simulink model "MAIN_V4"  (R2022a)
settings: Solver=VariableStepAuto  StartTime=0.0  StopTime=10  RelTol=1e-3
undefined symbols (not defined in the file): angDrag, c_Fuel, CM_FUEL_b, cmFuel_cmL, g, k_Fuel, KX, KY, L_TV, linDrag, m_dot, m_iFuel, VRfromNED_cordT, W_LANDER
libraries: matrix_library x4, slpidlib x1, dspsrcs4 x1, shared6dof x1, aerolibanim x1, simulink_extras x1, vrlib x1
settings Model: Creator=josepfamador  LastModifiedBy=Siste
settings DebuggingCC: UnconnectedInputMsg=warning  UnconnectedOutputMsg=warning  UnconnectedLineMsg=warning
settings RTWCC: DLArmComputeVersion=19.05

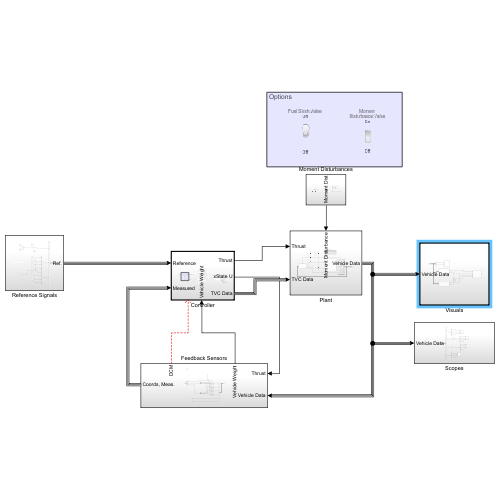
[thumbnail: Simulink's stored preview of the top-level diagram]
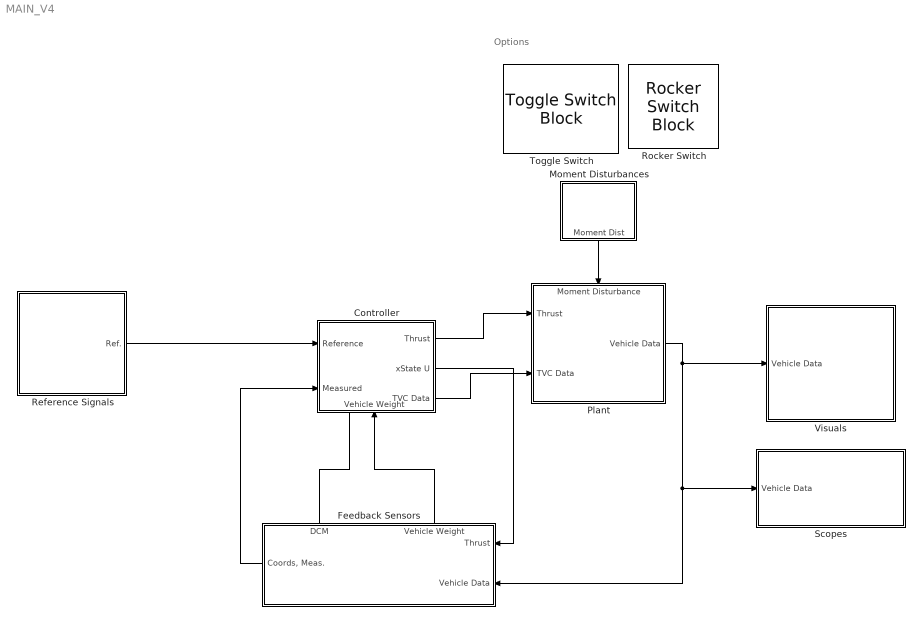
== system MAIN_V4 ==
  note: Options
  Controller : Subsystem  TreatAsAtomicUnit=on
      settings: PortSchema="{\"entries\":[{\"content\":{\"sides\":[{\"content\":{\"connectorIds\":[\"In1\",\"In2\"]},\"type\":\"ConnectorPlacement.EquallySpacedRectSide\",\"uuid\":\"a9e81047-82e7-465f-ace1-8f718b90561e\"},{\"content\":{\"connectorIds\":[\"Out1\",\"Out2\",\"Out3\"],\"side\":\"RIGHT\"},\"type\":\"ConnectorPlacement.EquallySpacedRectSide\",\"uuid\":\"e48627af-c2aa-4531-b804-41f44ff16765\"},{\"content\":{\"connectorIds\":[],\"side\":\"TOP\"},\"type\":\"ConnectorPlacement.EquallySpacedRectSide\",\"uuid\":\"f9e16229-b89b-4f8f-8331-a0f549979ea4\"},{\"content\":{\"connectorIds\":[\"In3\"],\"side\":\"BOTTOM\"},\"type\":\"ConnectorPlacement.EquallySpacedRectSide\",\"uuid\":\"04cdfde2-d4f0-49a2-8a73-ed462fcd7361\"}]},\"type\":\"ConnectorPlacement.EquallySpacedConnector\",\"uuid\":\"554d82b7-b70e-4d8b-909f-79f77f042d74\"}],\"packageUris\":[\"http://schema.mathworks.com/mf0/Connector/R2020b\"],\"version\":\"1.0\"}"
  Feedback Sensors : Subsystem
      settings: PortSchema="{\"entries\":[{\"content\":{\"sides\":[{\"content\":{\"connectorIds\":[\"In1\",\"In2\"]},\"type\":\"ConnectorPlacement.EquallySpacedRectSide\",\"uuid\":\"d175d4a2-8e54-4a4e-8022-790f4682ab06\"},{\"content\":{\"connectorIds\":[\"Out1\"],\"side\":\"RIGHT\"},\"type\":\"ConnectorPlacement.EquallySpacedRectSide\",\"uuid\":\"24f1a27c-01cc-42b0-9970-402e35771ac9\"},{\"content\":{\"connectorIds\":[\"Out2\",\"Out3\"],\"side\":\"TOP\"},\"type\":\"ConnectorPlacement.EquallySpacedRectSide\",\"uuid\":\"3106a051-6715-4641-97e9-232ad93b76cc\"}]},\"type\":\"ConnectorPlacement.EquallySpacedConnector\",\"uuid\":\"a13f3672-a567-4503-9f3c-ec2ff34e4e5d\"}],\"packageUris\":[\"http://schema.mathworks.com/mf0/Connector/R2020b\"],\"version\":\"1.0\"}"
  Moment Disturbances : Subsystem
  Plant : Subsystem
      settings: PortSchema="{\"entries\":[{\"content\":{\"sides\":[{\"content\":{\"connectorIds\":[\"In1\",\"In2\"]},\"type\":\"ConnectorPlacement.EquallySpacedRectSide\",\"uuid\":\"a9e81047-82e7-465f-ace1-8f718b90561e\"},{\"content\":{\"connectorIds\":[\"Out1\"],\"side\":\"RIGHT\"},\"type\":\"ConnectorPlacement.EquallySpacedRectSide\",\"uuid\":\"e48627af-c2aa-4531-b804-41f44ff16765\"},{\"content\":{\"connectorIds\":[\"In3\"],\"side\":\"TOP\"},\"type\":\"ConnectorPlacement.EquallySpacedRectSide\",\"uuid\":\"f9e16229-b89b-4f8f-8331-a0f549979ea4\"}]},\"type\":\"ConnectorPlacement.EquallySpacedConnector\",\"uuid\":\"554d82b7-b70e-4d8b-909f-79f77f042d74\"}],\"packageUris\":[\"http://schema.mathworks.com/mf0/Connector/R2020b\"],\"version\":\"1.0\"}"
  Reference Signals : Subsystem
  Rocker Switch : RockerSwitchBlock
      settings: Values={{'Off', 'On'}, [0 1]}
  Scopes : Subsystem
  Toggle Switch : ToggleSwitchBlock
      settings: Values={{'Off', 'On'}, [0 1]}
  Visuals : Subsystem  TreatAsAtomicUnit=on
  wires:
  Moment Disturbances/1(Moment Dist) -> Plant/3(Moment Disturbance)
  Plant/1(Vehicle Data) -> Scopes/1(Vehicle Data), Feedback Sensors/2(Vehicle Data), Visuals/1(Vehicle Data)
  Controller/1(Thrust) -> Plant/1(Thrust)
  Feedback Sensors/2(Vehicle Weight) -> Controller/3(Vehicle Weight)
  Feedback Sensors/3(DCM) -> ?
  Reference Signals/1(Ref.) -> Controller/1(Reference)
  Controller/2(xState U) -> Feedback Sensors/1(Thrust)
  Feedback Sensors/1("Coords, Meas.") -> Controller/2(Measured)
  Controller/3(TVC Data) -> Plant/2(TVC Data)

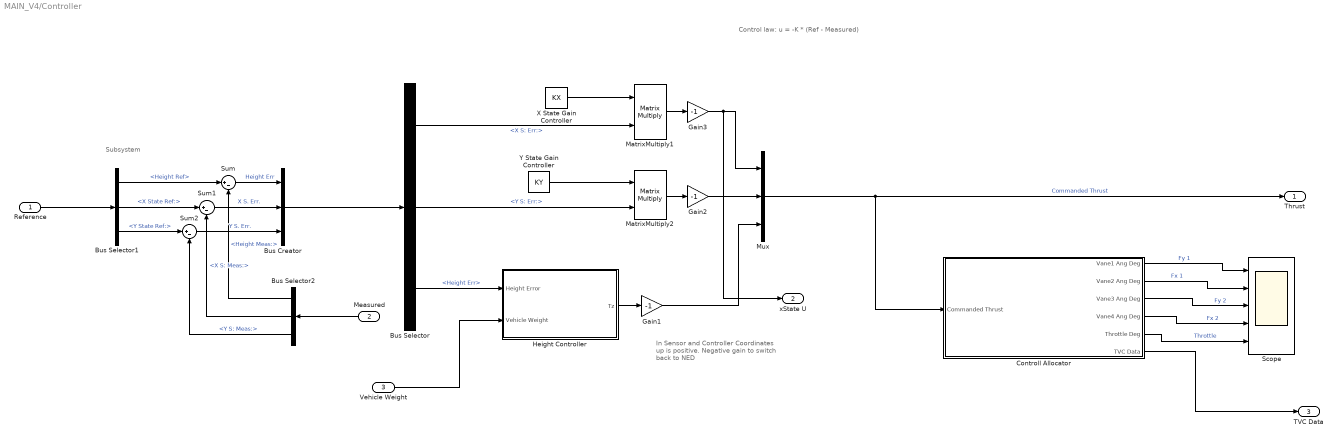
== system MAIN_V4/Controller ==
  note: Subsystem
  note: Control law: u = -K * (Ref - Measured)
  note: In Sensor and Controller Coordinates up is positive. Negative gain to switch back to NED
  Reference : Inport
  Measured : Inport  Port=2
  Vehicle Weight : Inport  Port=3
  Bus Creator : BusCreator  Inputs=3
  Bus Selector : BusSelector  OutputSignals=X S: Err:,Y S: Err:,Height Err
  Bus Selector1 : BusSelector  OutputSignals=Height Ref,X State Ref:,Y State Ref:
  Bus Selector2 : BusSelector  OutputSignals=Height Meas:,X S: Meas:,Y S: Meas:
  Controll Allocator : Subsystem
  Gain1 : Gain  Gain=-1
  Gain2 : Gain  Gain=-1
  Gain3 : Gain  Gain=-1
  Height Controller : Subsystem
  MatrixMultiply1 : Product  Multiplication=Matrix(*)
  MatrixMultiply2 : Product  Multiplication=Matrix(*)
  Mux : Mux  Inputs=3
  Scope : Scope  NumInputPorts=5
  Sum : Sum  Inputs=|+-
  Sum1 : Sum  Inputs=|+-
  Sum2 : Sum  Inputs=|+-
  X State Gain Controller : Constant  Value=KX  VectorParams1D=off
  Y State Gain Controller : Constant  Value=KY  VectorParams1D=off
  Thrust : Outport
  xState U : Outport  Port=2
  TVC Data : Outport  Port=3
  wires:
  Vehicle Weight/1 -> Height Controller/2(Vehicle Weight)
  Height Controller/1(Tz) -> Gain1/1
  Mux/1 -> Controll Allocator/1(Commanded Thrust), Thrust/1  "Commanded Thrust"
  Gain1/1 -> Mux/3
  X State Gain Controller/1 -> MatrixMultiply1/1
  Bus Selector/1 -> MatrixMultiply1/2  "<X S: Err:>"
  Y State Gain Controller/1 -> MatrixMultiply2/1
  Bus Selector/2 -> MatrixMultiply2/2  "<Y S: Err:>"
  Bus Selector/3 -> Height Controller/1(Height Error)  "<Height Err>"
  MatrixMultiply2/1 -> Gain2/1
  MatrixMultiply1/1 -> Gain3/1
  Gain2/1 -> Mux/2
  Gain3/1 -> xState U/1, Mux/1
  Controll Allocator/1(Vane1 Ang Deg) -> Scope/1  "Fy 1"
  Controll Allocator/2(Vane2 Ang Deg) -> Scope/2  "Fx 1"
  Controll Allocator/3(Vane3 Ang Deg) -> Scope/3  "Fy 2"
  Controll Allocator/4(Vane4 Ang Deg) -> Scope/4  "Fx 2"
  Controll Allocator/5(Throttle Deg) -> Scope/5  "Throttle"
  Reference/1 -> Bus Selector1/1
  Bus Selector2/2 -> Sum1/2  "<X S: Meas:>"
  Sum1/1 -> Bus Creator/2  "X S. Err."
  Sum2/1 -> Bus Creator/3  "Y S. Err."
  Bus Selector1/2 -> Sum1/1  "<X State Ref:>"
  Sum/1 -> Bus Creator/1  "Height Err"
  Bus Selector2/3 -> Sum2/2  "<Y S: Meas:>"
  Bus Selector1/3 -> Sum2/1  "<Y State Ref:>"
  Bus Selector1/1 -> Sum/1  "<Height Ref>"
  Bus Creator/1 -> Bus Selector/1
  Bus Selector2/1 -> Sum/2  "<Height Meas:>"
  Measured/1 -> Bus Selector2/1
  Controll Allocator/6(TVC Data) -> TVC Data/1

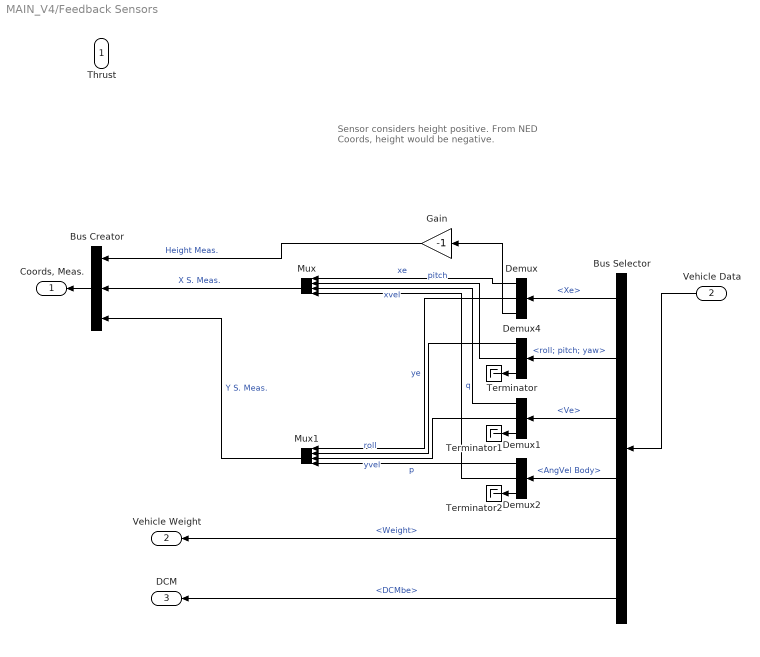
== system MAIN_V4/Feedback Sensors ==
  note: Sensor considers height positive.
      | From NED Coords, height would be negative.
  Thrust : Inport
  Vehicle Data : Inport  Port=2
  Bus Creator : BusCreator  Inputs=3
  Bus Selector : BusSelector  OutputSignals=Xe,roll; pitch; yaw,Ve,AngVel Body,Weight,DCMbe
  Demux{,1..2,4} (4 alike) : Demux  Outputs=3
  Gain : Gain  Gain=-1
  Mux : Mux
  Mux1 : Mux
  Terminator : Terminator
  Terminator1 : Terminator
  Terminator2 : Terminator
  "Coords, Meas." : Outport
  Vehicle Weight : Outport  Port=2
  DCM : Outport  Port=3
  wires:
  Vehicle Data/1 -> Bus Selector/1
  Bus Selector/1 -> Demux/1  "<Xe>"
  Bus Selector/2 -> Demux4/1  "<roll; pitch; yaw>"
  Demux/3 -> Gain/1
  Demux/1 -> Mux/1  "xe"
  Demux/2 -> Mux1/1  "ye"
  Gain/1 -> Bus Creator/1  "Height Meas."
  Bus Selector/5 -> Vehicle Weight/1  "<Weight>"
  Bus Selector/6 -> DCM/1  "<DCMbe>"
  Demux4/2 -> Mux/2  "pitch"
  Bus Selector/4 -> Demux2/1  "<AngVel Body>"
  Bus Selector/3 -> Demux1/1  "<Ve>"
  Demux1/1 -> Mux/3  "xvel"
  Demux2/2 -> Mux/4  "q"
  Mux/1 -> Bus Creator/2  "X S. Meas."
  Mux1/1 -> Bus Creator/3  "Y S. Meas."
  Demux4/1 -> Mux1/2  "roll"
  Demux1/2 -> Mux1/3  "yvel"
  Demux2/1 -> Mux1/4  "p"
  Demux4/3 -> Terminator/1
  Demux1/3 -> Terminator1/1
  Demux2/3 -> Terminator2/1
  Bus Creator/1 -> "Coords, Meas."/1

== system MAIN_V4/Moment Disturbances ==
  Demux : Demux  Outputs=3
  Disturbance Vector : Subsystem
  Moment Disturbance : Constant  Value=0
  Scope : Scope  NumInputPorts=3
  Slider : SliderBlock  ScaleMax=20
  Moment Dist : Outport
  wires:
  Disturbance Vector/1(Out1) -> Demux/1, Moment Dist/1
  Moment Disturbance/1 -> Disturbance Vector/Enable
  Demux/1 -> Scope/1
  Demux/2 -> Scope/2
  Demux/3 -> Scope/3

== system MAIN_V4/Plant ==
  note: Coordinate Frame used.
      | X
      | Into the Screen. Away from Observer
      |
      | Y
      | Right Of Screen. Observer's Right
      |
      | Z
      | Down to ground. Observer's Ground
  Thrust : Inport
  TVC Data : Inport  Port=2
  Moment Disturbance : Inport  Port=3
  6DOF (Euler Angles) : shared6dof/6DOF (Euler Angles)  units=Metric (MKS)  mtype=Fixed  rep=Euler Angles  xme_0=[0 0 0]  Vm_0=[0 0 0]  eul_0=[0 0 0]  pm_0=[0 0 0]  mass_0=M_lander  mass_e=0.5  mass_f=2.0  inertia=I  inertia_e=eye(3)  inertia_f=2*eye(3)  k_quat=1.0  vre_flag=on  abi_flag=off  aMode=0  xme_statename=''  Vm_statename=''  eul_statename=''  quat_statename=''  pm_statename=''  mass_statename=''
      settings: SourceProductBaseCode=AE,PW,DR,MT,VE
  Bus Creator1 : BusCreator  Inputs=11
  Forces and Moments : Subsystem
      settings: PortSchema="{\"entries\":[{\"content\":{\"sides\":[{\"content\":{\"connectorIds\":[\"In1\"]},\"type\":\"ConnectorPlacement.EquallySpacedRectSide\",\"uuid\":\"828f15e3-cbad-415f-85fb-ba6a8e0cd3b9\"},{\"content\":{\"connectorIds\":[\"Out1\",\"Out2\",\"Out3\"],\"side\":\"RIGHT\"},\"type\":\"ConnectorPlacement.EquallySpacedRectSide\",\"uuid\":\"5000816a-8e0b-4f65-bf77-7d05076903d9\"},{\"content\":{\"connectorIds\":[\"In2\"],\"side\":\"TOP\"},\"type\":\"ConnectorPlacement.EquallySpacedRectSide\",\"uuid\":\"57f53c13-0af9-4c97-9cf0-1ba4f356b699\"}]},\"type\":\"ConnectorPlacement.EquallySpacedConnector\",\"uuid\":\"7fdc047f-04f4-4b62-afef-380f9e9b929b\"}],\"packageUris\":[\"http://schema.mathworks.com/mf0/Connector/R2020b\"],\"version\":\"1.0\"}"
  Sum : Sum  Inputs=++|
  Sum1 : Sum  Inputs=++|
  Vehicle Data : Outport
  wires:
  6DOF (Euler Angles)/7 -> Bus Creator1/7  "AngAcc body"
  6DOF (Euler Angles)/3 -> Bus Creator1/3  "roll, pitch, yaw"
  Sum/1 -> 6DOF (Euler Angles)/1
  Thrust/1 -> Sum/1, Forces and Moments/2(Thrust), Bus Creator1/10  "Thrust"
  6DOF (Euler Angles)/4 -> Bus Creator1/4  "DCMbe"
  Forces and Moments/1(SumF) -> Sum/2
  Forces and Moments/2(Moments) -> Sum1/2
  6DOF (Euler Angles)/6 -> Bus Creator1/6  "AngVel Body"
  6DOF (Euler Angles)/1 -> Bus Creator1/1  "Ve"
  6DOF (Euler Angles)/2 -> Bus Creator1/2  "Xe"
  6DOF (Euler Angles)/5 -> Bus Creator1/5  "Vb"
  6DOF (Euler Angles)/8 -> Bus Creator1/8  "Acc Body"
  Bus Creator1/1 -> Forces and Moments/1(Vehicle Data), Vehicle Data/1
  Sum1/1 -> 6DOF (Euler Angles)/2
  Moment Disturbance/1 -> Sum1/1
  Forces and Moments/3(Total Weight) -> Bus Creator1/9  "Weight"
  TVC Data/1 -> Bus Creator1/11  "TVC Data"

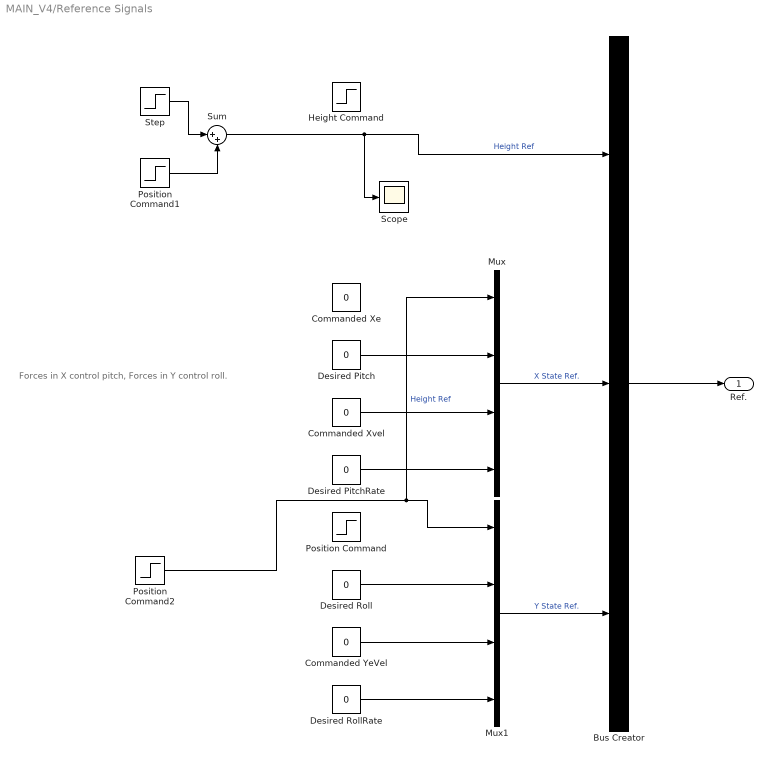
== system MAIN_V4/Reference Signals ==
  note: Forces in X control pitch, Forces in Y control roll.
  Bus Creator : BusCreator  Inputs=3
  Commanded Xe : Constant  Value=0
  Commanded Xvel : Constant  Value=0
  Commanded YeVel : Constant  Value=0
  Desired Pitch : Constant  Value=0
  Desired PitchRate : Constant  Value=0
  Desired Roll : Constant  Value=0
  Desired RollRate : Constant  Value=0
  Height Command : Step  SampleTime=0
  Mux : Mux
  Mux1 : Mux
  Position Command : Step  Time=3  SampleTime=0
  Position Command1 : Step  Time=0.5  SampleTime=0
  Position Command2 : Step  SampleTime=0
  Scope : Scope
  Step : Step  Time=6  After=-1  SampleTime=0
  Sum : Sum  Inputs=|++
  Ref. : Outport
  wires:
  Sum/1 -> Scope/1, Bus Creator/1  "Height Ref"
  Desired PitchRate/1 -> Mux/4
  Commanded Xvel/1 -> Mux/3
  Desired Pitch/1 -> Mux/2
  Mux/1 -> Bus Creator/2  "X State Ref."
  Desired Roll/1 -> Mux1/2
  Commanded YeVel/1 -> Mux1/3
  Desired RollRate/1 -> Mux1/4
  Mux1/1 -> Bus Creator/3  "Y State Ref."
  Bus Creator/1 -> Ref./1
  Position Command1/1 -> Sum/2
  Step/1 -> Sum/1
  Position Command2/1 -> Mux/1, Mux1/1  "Height Ref"

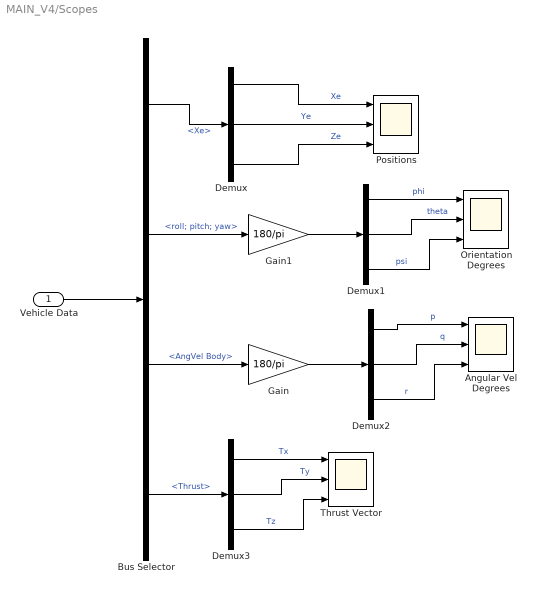
== system MAIN_V4/Scopes ==
  Vehicle Data : Inport
  Angular Vel Degrees : Scope  NumInputPorts=3
  Bus Selector : BusSelector  OutputSignals=Xe,roll; pitch; yaw,AngVel Body,Thrust
  Demux{,1..3} (4 alike) : Demux  Outputs=3
  Gain : Gain  Gain=180/pi
  Gain1 : Gain  Gain=180/pi
  Orientation Degrees : Scope  NumInputPorts=3
  Positions : Scope  NumInputPorts=3
  Thrust Vector : Scope  NumInputPorts=3
  wires:
  Vehicle Data/1 -> Bus Selector/1
  Bus Selector/1 -> Demux/1  "<Xe>"
  Bus Selector/3 -> Gain/1  "<AngVel Body>"
  Bus Selector/2 -> Gain1/1  "<roll; pitch; yaw>"
  Demux/2 -> Positions/2  "Ye"
  Demux/1 -> Positions/1  "Xe"
  Demux/3 -> Positions/3  "Ze"
  Demux1/1 -> Orientation Degrees/1  "phi"
  Demux1/2 -> Orientation Degrees/2  "theta"
  Demux1/3 -> Orientation Degrees/3  "psi"
  Demux2/2 -> Angular Vel Degrees/2  "q"
  Demux2/1 -> Angular Vel Degrees/1  "p"
  Demux2/3 -> Angular Vel Degrees/3  "r"
  Bus Selector/4 -> Demux3/1  "<Thrust>"
  Demux3/1 -> Thrust Vector/1  "Tx"
  Demux3/2 -> Thrust Vector/2  "Ty"
  Demux3/3 -> Thrust Vector/3  "Tz"
  Gain/1 -> Demux2/1
  Gain1/1 -> Demux1/1

== system MAIN_V4/Visuals ==
  Vehicle Data : Inport
  6DoF Animation1 : aerolibanim/6DoF Animation  u1=[-5 5 -5 5 0 4]  u2=0.1  u3=1  u4=[0 0 -1]  u5=Fixed position  u6=[-10 0 0]  u7=45  u8=off
  Bus Selector : BusSelector  OutputSignals=Xe,roll; pitch; yaw
  Coordinate Transforms : Subsystem
  Coordinate Transforms1 : Subsystem
  Sum1 : Sum  Inputs=|++
  VR Sink : vrlib/VR Sink  InstantiateOnLoad=on  SampleTime=0.016  ViewEnable=on  RemoteChange=off  RemoteView=off  FieldsWritten=Lander.rotation.4.1.1.double#Lander.translation.3.1.1.double#ThrustVector.rotation.4.1.1.double#ThrustVector.translation.3.1.1.double  WorldFileName=vrsinkstuff\v7b.x3d  AutoView=off  VideoDimensions=[200 320]  AllowVariableSize=off
  wires:
  Bus Selector/1 -> 6DoF Animation1/1  "<Xe>"
  Bus Selector/2 -> 6DoF Animation1/2  "<roll; pitch; yaw>"
  Vehicle Data/1 -> Bus Selector/1, Coordinate Transforms/1(Vehicle Data), Coordinate Transforms1/1(Vehicle Data)
  Coordinate Transforms/2(VR Translation) -> Sum1/2, VR Sink/2  "Lander Translation"
  Coordinate Transforms1/2(TV Translation) -> Sum1/1
  Coordinate Transforms/1(VR Rotation) -> VR Sink/1  "Lander Rotation"
  Sum1/1 -> VR Sink/4  "Thrust Vector Translation"
  Coordinate Transforms1/1(VR Rotation) -> VR Sink/3  "Thrust Vector Rotation"

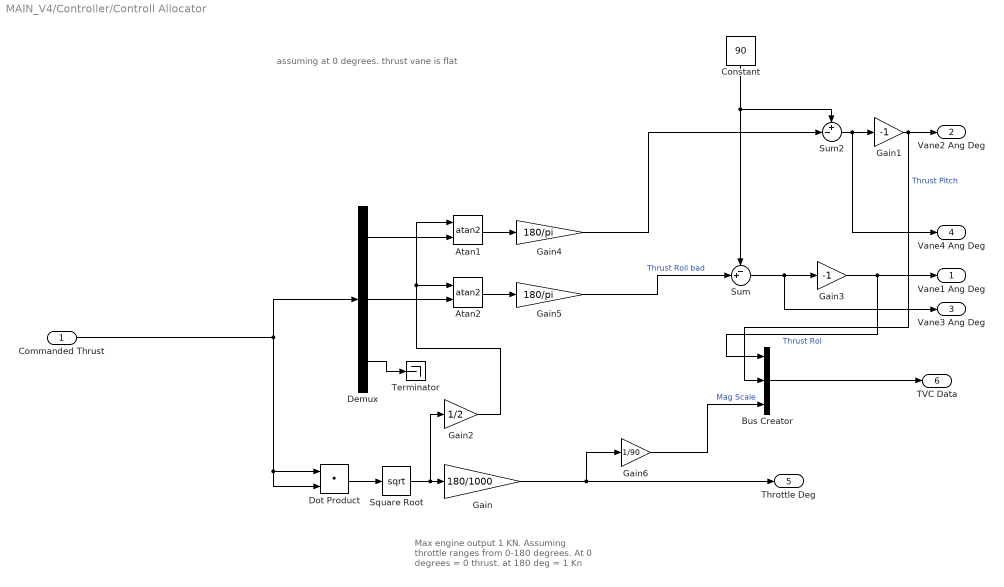
== system MAIN_V4/Controller/Controll Allocator ==
  note: assuming at 0 degrees. thrust vane is flat
  note: Max engine output 1 KN. Assuming throttle ranges from 0-180 degrees. At 0 degrees = 0 thrust. at 180 deg = 1 Kn
  Commanded Thrust : Inport
  Atan1 : Trigonometry  Operator=atan2
  Atan2 : Trigonometry  Operator=atan2
  Bus Creator : BusCreator  Inputs=3
  Constant : Constant  Value=90
  Demux : Demux  Outputs=3
  Dot Product : DotProduct  OutDataTypeStr=Inherit: Inherit via internal rule
  Gain : Gain  Gain=180/1000
  Gain1 : Gain  Gain=-1
  Gain2 : Gain  Gain=1/2
  Gain3 : Gain  Gain=-1
  Gain4 : Gain  Gain=180/pi
  Gain5 : Gain  Gain=180/pi
  Gain6 : Gain  Gain=1/90
  Square Root : Sqrt
  Sum : Sum  Inputs=-+|
  Sum2 : Sum  Inputs=+-|
  Terminator : Terminator
  Vane1 Ang Deg : Outport
  Vane2 Ang Deg : Outport  Port=2
  Vane3 Ang Deg : Outport  Port=3
  Vane4 Ang Deg : Outport  Port=4
  Throttle Deg : Outport  Port=5
  TVC Data : Outport  Port=6
  wires:
  Commanded Thrust/1 -> Demux/1, Dot Product/1, Dot Product/2
  Dot Product/1 -> Square Root/1
  Square Root/1 -> Gain2/1, Gain/1
  Gain/1 -> Gain6/1, Throttle Deg/1
  Demux/3 -> Terminator/1
  Demux/2 -> Atan2/2
  Gain2/1 -> Atan2/1, Atan1/1
  Atan2/1 -> Gain5/1
  Constant/1 -> Sum/1, Sum2/1
  Sum/1 -> Vane3 Ang Deg/1, Gain3/1
  Demux/1 -> Atan1/2
  Atan1/1 -> Gain4/1
  Sum2/1 -> Vane4 Ang Deg/1, Gain1/1
  Gain4/1 -> Sum2/2
  Gain5/1 -> Sum/2  "Thrust Roll bad"
  Gain1/1 -> Bus Creator/2, Vane2 Ang Deg/1  "Thrust Pitch"
  Gain3/1 -> Vane1 Ang Deg/1, Bus Creator/1  "Thrust Rol"
  Gain6/1 -> Bus Creator/3  "Mag Scale"
  Bus Creator/1 -> TVC Data/1

== system MAIN_V4/Controller/Height Controller ==
  Height Error : Inport
  Vehicle Weight : Inport  Port=2
  Dot Product : DotProduct  OutDataTypeStr=Inherit: Inherit via internal rule
  PID Controller : slpidlib/PID Controller  Controller=PID  Form=Parallel  TimeDomain=Discrete-time  UseExternalTs=off  SampleTime=1/50  IntegratorMethod=Forward Euler  FilterMethod=Forward Euler  ControllerParametersSource=internal  P=0.286875183119282  I=0.000955327447568306  UseKiTs=off  D=19.1392868198824  N=39.4808387317057  UseFilter=on  TunerSelectOption=Transfer Function Based (PID Tuner App)  InitialConditionSource=internal  InitialConditionForIntegrator=0  InitialConditionForFilter=0  DifferentiatorICPrevScaledInput=0  ExternalReset=none  TrackingMode=off  Kt=1  LimitOutput=on  SatLimitsSource=internal  UpperSaturationLimit=500  LowerSaturationLimit=-500  LinearizeAsGain=on  AntiWindupMode=none  Kb=1  POutMin=[]  POutMax=[]  IOutMin=[]  IOutMax=[]  DOutMin=[]  DOutMax=[]  NOutMin=[]  NOutMax=[]  SumOutMin=[]  SumOutMax=[]  SaturationOutMin=[]  SaturationOutMax=[]  PParamMin=[]  PParamMax=[]  IParamMin=[]  IParamMax=[]  DParamMin=[]  DParamMax=[]  NParamMin=[]  NParamMax=[]  KbParamMin=[]  KbParamMax=[]  KtParamMin=[]  KtParamMax=[]  KbOutMin=[]  KbOutMax=[]  KtOutMin=[]  KtOutMax=[]  IntegratorOutMin=[]  IntegratorOutMax=[]  FilterOutMin=[]  FilterOutMax=[]  SumI1OutMin=[]  SumI1OutMax=[]  SumI2OutMin=[]  SumI2OutMax=[]  SumI3OutMin=[]  SumI3OutMax=[]  SumI4OutMin=[]  SumI4OutMax=[]  SumDOutMin=[]  SumDOutMax=[]  DifferentiatorOutMin=[]  DifferentiatorOutMax=[]  FilterDiffOutCoefMin=[]  FilterDiffOutCoefMax=[]  ReciprocalOutMin=[]  ReciprocalOutMax=[]  SumDenOutMin=[]  SumDenOutMax=[]  SumNumOutMin=[]  SumNumOutMax=[]  DivideOutMin=[]  DivideOutMax=[]  UdiffTsProdOutMin=[]  UdiffTsProdOutMax=[]  NTsProdOutMin=[]  NTsProdOutMax=[]  UintegralTsProdOutMin=[]  UintegralTsProdOutMax=[]  UngainTsProdOutMin=[]  UngainTsProdOutMax=[]  IntegratorContinuousStateAttributes=''  IntegratorStateMustResolveToSignalObject=off  IntegratorRTWStateStorageClass=Auto  FilterContinuousStateAttributes=''  FilterStateMustResolveToSignalObject=off  FilterRTWStateStorageClass=Auto  ParallelPVariant=InternalParameters  IdealPVariant=Disabled  IVariant=InternalParameters  DVariant=InternalParameters  IntegratorVariant=Discrete  SatVariant=Enabled  AWVariant=Passthrough  PCopyVariant=Disabled  TRVariant=Disabled  FdbkBlocksVariant=Forward  IdealPFdbkVariant=Disabled  SatFdbkVariant=Disabled  DerivativeFilterVariant=ForwardEulerFilter  NVariant=InternalParameters  NCopyVariant=Disabled  FilterICVariant=InternalICsFilter  IntegratorICVariant=InternalICs  ExternalResetVariant=Disabled  TRSumVariant=Passthrough  SumFdbkVariant=Disabled  SumVariant=Sum_PID  TsampFilterVariant=InternalTs  TsampNgainVariant=Passthrough  TsampIntegralVariant=Passthrough  ExternalSaturationOutDataTypeStr=Inherit: Same as second input  aMode=0
  Square Root : Sqrt
  Sum : Sum  Inputs=++|
  Tz : Outport
  wires:
  Height Error/1 -> PID Controller/1
  Vehicle Weight/1 -> Dot Product/1, Dot Product/2
  Dot Product/1 -> Square Root/1
  PID Controller/1 -> Sum/2  "Thrust Difference"
  Square Root/1 -> Sum/1
  Sum/1 -> Tz/1

== system MAIN_V4/Moment Disturbances/Disturbance Vector ==
  Enable : EnablePort
  Constant : Constant  Value=0
  Discrete Impulse : dspsrcs4/Discrete  Impulse  Delay=200  SampleTime=0.01  FrameSample=1  OutputFrames=off  dataType=double  isSigned=on  wordLen=16  udDataType=sfix(16)  fracBitsMode=Best precision  numFracBits=15  OutDataTypeStr=double  LastOutDataTypeStr=double
  Impulse Magnitude (Newtons) : Gain  Gain=20
  Mux : Mux  Inputs=3
  Out1 : Outport
  wires:
  Mux/1 -> Out1/1
  Discrete Impulse/1 -> Impulse Magnitude (Newtons)/1
  Constant/1 -> Mux/3
  Impulse Magnitude (Newtons)/1 -> Mux/2, Mux/1

== system MAIN_V4/Plant/Forces and Moments ==
  Vehicle Data : Inport
  Thrust : Inport  Port=2
  Forces Body Fixed Frame : Subsystem  TreatAsAtomicUnit=on
      settings: PortSchema="{\"entries\":[{\"content\":{\"sides\":[{\"content\":{\"connectorIds\":[\"In1\"]},\"type\":\"ConnectorPlacement.EquallySpacedRectSide\",\"uuid\":\"828f15e3-cbad-415f-85fb-ba6a8e0cd3b9\"},{\"content\":{\"connectorIds\":[\"Out1\",\"Out2\"],\"side\":\"RIGHT\"},\"type\":\"ConnectorPlacement.EquallySpacedRectSide\",\"uuid\":\"5000816a-8e0b-4f65-bf77-7d05076903d9\"},{\"content\":{\"connectorIds\":[],\"side\":\"TOP\"},\"type\":\"ConnectorPlacement.EquallySpacedRectSide\",\"uuid\":\"57f53c13-0af9-4c97-9cf0-1ba4f356b699\"},{\"content\":{\"connectorIds\":[\"Out3\",\"Out4\"],\"side\":\"BOTTOM\"},\"type\":\"ConnectorPlacement.EquallySpacedRectSide\",\"uuid\":\"07d00598-10e4-47df-ac26-33e6f3a9eead\"}]},\"type\":\"ConnectorPlacement.EquallySpacedConnector\",\"uuid\":\"7fdc047f-04f4-4b62-afef-380f9e9b929b\"}],\"packageUris\":[\"http://schema.mathworks.com/mf0/Connector/R2020b\"],\"version\":\"1.0\"}"
  Moments Body Fixed : Subsystem
      settings: PortSchema="{\"entries\":[{\"content\":{\"sides\":[{\"content\":{\"connectorIds\":[\"In1\",\"In2\"]},\"type\":\"ConnectorPlacement.EquallySpacedRectSide\",\"uuid\":\"bf632890-9061-4ebf-b839-17051433f7d2\"},{\"content\":{\"connectorIds\":[\"Out1\"],\"side\":\"RIGHT\"},\"type\":\"ConnectorPlacement.EquallySpacedRectSide\",\"uuid\":\"d3255547-983f-46fe-8ffa-de3f6c331a2a\"},{\"content\":{\"connectorIds\":[\"In3\",\"In4\"],\"side\":\"TOP\"},\"type\":\"ConnectorPlacement.EquallySpacedRectSide\",\"uuid\":\"18f3806f-6d56-407f-aadd-d25baf8c86b7\"}]},\"type\":\"ConnectorPlacement.EquallySpacedConnector\",\"uuid\":\"1b0eb8e4-97ea-4203-914f-8b852a07c841\"}],\"packageUris\":[\"http://schema.mathworks.com/mf0/Connector/R2020b\"],\"version\":\"1.0\"}"
  SumF : Outport
  Moments : Outport  Port=2
  Total Weight : Outport  Port=3
  wires:
  Forces Body Fixed Frame/1(SumF) -> SumF/1
  Moments Body Fixed/1(Moment) -> Moments/1
  Forces Body Fixed Frame/3(Fuel Slosh Vector) -> Moments Body Fixed/2(Slosh)
  Thrust/1 -> Moments Body Fixed/1(Thrust)
  Forces Body Fixed Frame/4(Weight Fuel (Body Fixed)) -> Moments Body Fixed/3(Weight Body Fixed)
  Vehicle Data/1 -> Moments Body Fixed/4(Vehicle Data), Forces Body Fixed Frame/1(Vehicle Data)
  Forces Body Fixed Frame/2(Total Weight) -> Total Weight/1

== system MAIN_V4/Visuals/Coordinate Transforms ==
  Vehicle Data : Inport
  Bus Selector : BusSelector  OutputSignals=Xe,roll; pitch; yaw
  Constant : Constant  Value=VRfromNED_cordT
  Generalized Principle Axis and Angle of Rotation : MATLAB Function  TreatAsAtomicUnit=on
  MatrixMultiply : Product  Multiplication=Matrix(*)
  NED Euler to VR Euler : MATLAB Function  TreatAsAtomicUnit=on
  VR Rotation : Outport
  VR Translation : Outport  Port=2
  wires:
  Vehicle Data/1 -> Bus Selector/1
  Constant/1 -> MatrixMultiply/1
  Bus Selector/1 -> MatrixMultiply/2  "<Xe>"
  Bus Selector/2 -> NED Euler to VR Euler/1(eu)  "<roll; pitch; yaw>"
  NED Euler to VR Euler/1(C) -> Generalized Principle Axis and Angle of Rotation/1(RotMat)
  MatrixMultiply/1 -> VR Translation/1
  Generalized Principle Axis and Angle of Rotation/1(VRVec) -> VR Rotation/1

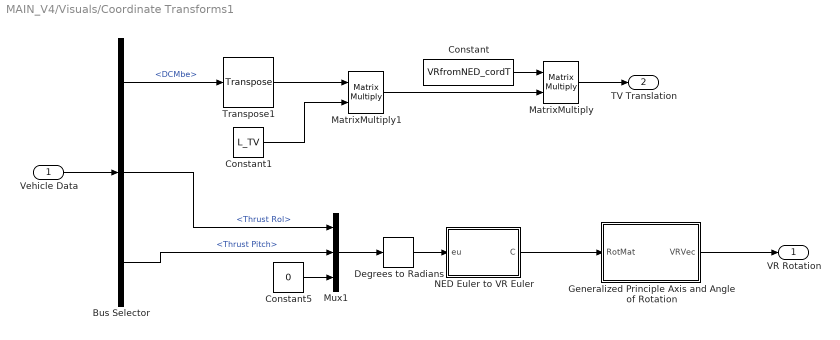
== system MAIN_V4/Visuals/Coordinate Transforms1 ==
  Vehicle Data : Inport
  Bus Selector : BusSelector  OutputSignals=DCMbe,TVC Data.Thrust Rol,TVC Data.Thrust Pitch
  Constant : Constant  Value=VRfromNED_cordT
  Constant1 : Constant  Value=L_TV
  Constant5 : Constant  Value=0
  Degrees to Radians : simulink_extras/Transformations/Degrees to Radians
  Generalized Principle Axis and Angle of Rotation : MATLAB Function  TreatAsAtomicUnit=on
  MatrixMultiply : Product  Multiplication=Matrix(*)
  MatrixMultiply1 : Product  Multiplication=Matrix(*)
  Mux1 : Mux  Inputs=3
  NED Euler to VR Euler : MATLAB Function  TreatAsAtomicUnit=on
  Transpose1 : matrix_library/Transpose
      settings: SourceProductBaseCode=SL
  VR Rotation : Outport
  TV Translation : Outport  Port=2
  wires:
  Vehicle Data/1 -> Bus Selector/1
  NED Euler to VR Euler/1(C) -> Generalized Principle Axis and Angle of Rotation/1(RotMat)
  Generalized Principle Axis and Angle of Rotation/1(VRVec) -> VR Rotation/1
  Bus Selector/1 -> Transpose1/1  "<DCMbe>"
  Transpose1/1 -> MatrixMultiply1/1
  Constant1/1 -> MatrixMultiply1/2
  Constant/1 -> MatrixMultiply/1
  MatrixMultiply1/1 -> MatrixMultiply/2
  MatrixMultiply/1 -> TV Translation/1
  Constant5/1 -> Mux1/3
  Bus Selector/2 -> Mux1/1  "<Thrust Rol>"
  Mux1/1 -> Degrees to Radians/1
  Degrees to Radians/1 -> NED Euler to VR Euler/1(eu)
  Bus Selector/3 -> Mux1/2  "<Thrust Pitch>"

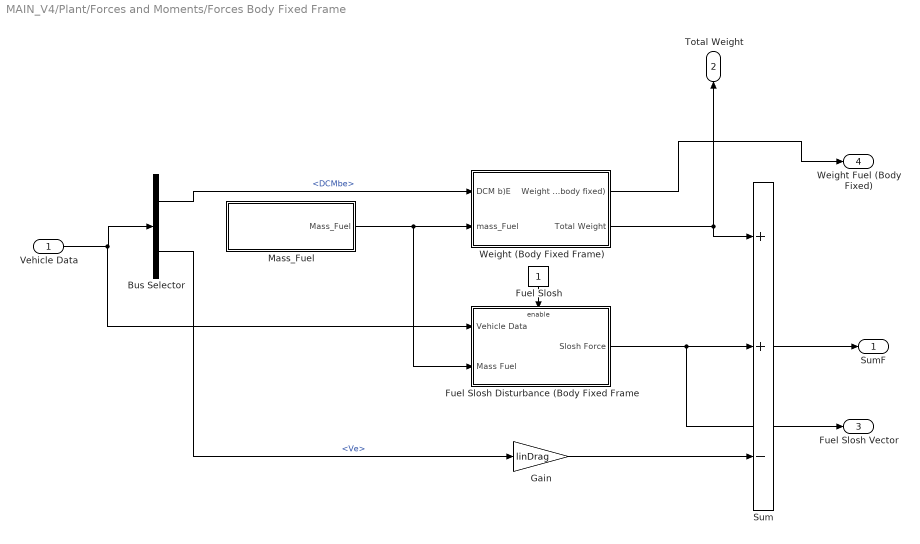
== system MAIN_V4/Plant/Forces and Moments/Forces Body Fixed Frame ==
  Vehicle Data : Inport
  Bus Selector : BusSelector  OutputSignals=DCMbe,Ve
  Fuel Slosh : Constant
  Fuel Slosh Disturbance (Body Fixed Frame : Subsystem
  Gain : Gain  Gain=linDrag
  Mass_Fuel : Subsystem
  Sum : Sum  Inputs=++-
  Weight (Body Fixed Frame) : Subsystem
  SumF : Outport
  Total Weight : Outport  Port=2
  Fuel Slosh Vector : Outport  Port=3
  Weight Fuel (Body Fixed) : Outport  Port=4
  wires:
  Mass_Fuel/1(Mass_Fuel) -> Fuel Slosh Disturbance (Body Fixed Frame/2(Mass Fuel), Weight (Body Fixed Frame)/2(mass_Fuel)
  Weight (Body Fixed Frame)/2(Total Weight) -> Total Weight/1, Sum/1
  Fuel Slosh Disturbance (Body Fixed Frame/1(Slosh Force) -> Fuel Slosh Vector/1, Sum/2
  Sum/1 -> SumF/1
  Fuel Slosh/1 -> Fuel Slosh Disturbance (Body Fixed Frame/Enable
  Weight (Body Fixed Frame)/1(Weight Fuel (body fixed)) -> Weight Fuel (Body Fixed)/1
  Vehicle Data/1 -> Fuel Slosh Disturbance (Body Fixed Frame/1(Vehicle Data), Bus Selector/1
  Bus Selector/1 -> Weight (Body Fixed Frame)/1(DCM b)E)  "<DCMbe>"
  Bus Selector/2 -> Gain/1  "<Ve>"
  Gain/1 -> Sum/3

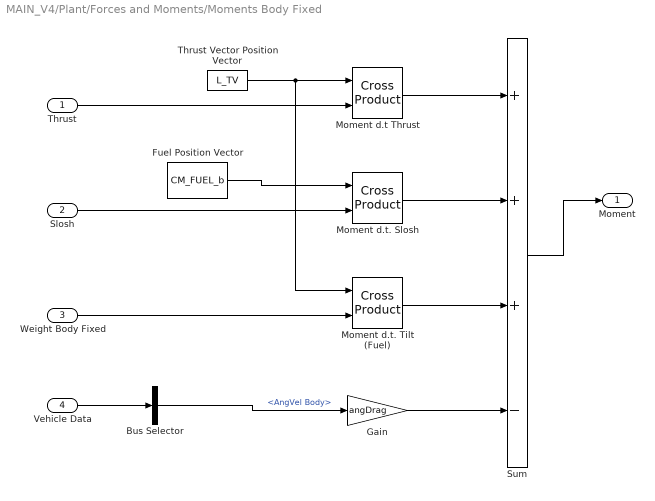
== system MAIN_V4/Plant/Forces and Moments/Moments Body Fixed ==
  Thrust : Inport
  Slosh : Inport  Port=2
  Weight Body Fixed : Inport  Port=3
  Vehicle Data : Inport  Port=4
  Bus Selector : BusSelector  OutputSignals=AngVel Body
  Fuel Position Vector : Constant  Value=CM_FUEL_b
  Gain : Gain  Gain=angDrag
  Moment d.t Thrust : matrix_library/Cross Product
      settings: SourceProductBaseCode=SL
  Moment d.t. Slosh : matrix_library/Cross Product
      settings: SourceProductBaseCode=SL
  Moment d.t. Tilt (Fuel) : matrix_library/Cross Product
      settings: SourceProductBaseCode=SL
  Sum : Sum  Inputs=+++-
  Thrust Vector Position Vector : Constant  Value=L_TV
  Moment : Outport
  wires:
  Thrust/1 -> Moment d.t Thrust/2
  Thrust Vector Position Vector/1 -> Moment d.t. Tilt (Fuel)/1, Moment d.t Thrust/1
  Slosh/1 -> Moment d.t. Slosh/2
  Fuel Position Vector/1 -> Moment d.t. Slosh/1
  Weight Body Fixed/1 -> Moment d.t. Tilt (Fuel)/2
  Moment d.t. Tilt (Fuel)/1 -> Sum/3
  Moment d.t. Slosh/1 -> Sum/2
  Moment d.t Thrust/1 -> Sum/1
  Sum/1 -> Moment/1
  Vehicle Data/1 -> Bus Selector/1
  Bus Selector/1 -> Gain/1  "<AngVel Body>"
  Gain/1 -> Sum/4

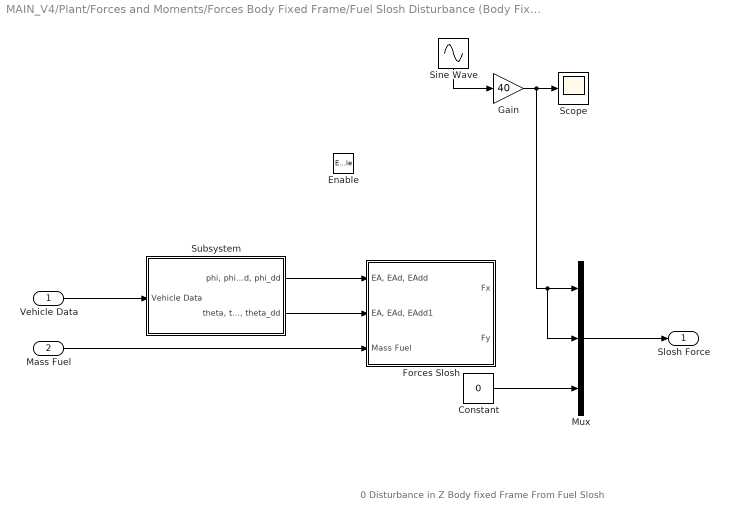
== system MAIN_V4/Plant/Forces and Moments/Forces Body Fixed Frame/Fuel Slosh Disturbance (Body Fixed Frame ==
  note: 0 Disturbance in Z Body fixed Frame From Fuel Slosh
  Vehicle Data : Inport
  Mass Fuel : Inport  Port=2
  Enable : EnablePort
  Constant : Constant  Value=0
  Forces Slosh : Subsystem
  Gain : Gain  Gain=40
  Mux : Mux  Inputs=3
  Scope : Scope
  Sine Wave : Sin  Frequency=18  SampleTime=0
  Subsystem : Subsystem
  Slosh Force : Outport
  wires:
  Subsystem/1("phi, phi_d, phi_dd") -> Forces Slosh/1("EA, EAd, EAdd")
  Subsystem/2("theta, theta_d, theta_dd") -> Forces Slosh/2("EA, EAd, EAdd1")
  Mass Fuel/1 -> Forces Slosh/3(Mass Fuel)
  Constant/1 -> Mux/3
  Mux/1 -> Slosh Force/1
  Vehicle Data/1 -> Subsystem/1(Vehicle Data)
  Sine Wave/1 -> Gain/1
  Gain/1 -> Mux/2, Mux/1, Scope/1

== system MAIN_V4/Plant/Forces and Moments/Forces Body Fixed Frame/Mass_Fuel ==
  note: m_dot set to 0
  Clock : Clock
  Sum : Sum  Inputs=+-|
  mass_burn_rate : Gain  Gain=m_dot
  mass_intial_fuel : Constant  Value=m_iFuel
  Mass_Fuel : Outport
  wires:
  mass_burn_rate/1 -> Sum/2
  Sum/1 -> Mass_Fuel/1
  mass_intial_fuel/1 -> Sum/1
  Clock/1 -> mass_burn_rate/1

== system MAIN_V4/Plant/Forces and Moments/Forces Body Fixed Frame/Weight (Body Fixed Frame) ==
  note: Forces In Earth Frame
  DCM b)E : Inport
  mass_Fuel : Inport  Port=2
  MatrixMultiply : Product  Multiplication=Matrix(*)
  MatrixMultiply1 : Product  Multiplication=Matrix(*)
  Sum : Sum
  Weigh_lander : Constant  Value=W_LANDER
  Weight_Fuel : Subsystem  TreatAsAtomicUnit=on
  Weight Fuel (body fixed) : Outport
  Total Weight : Outport  Port=2
  wires:
  mass_Fuel/1 -> Weight_Fuel/1(mass_Fuel)
  DCM b)E/1 -> MatrixMultiply1/1, MatrixMultiply/1
  MatrixMultiply1/1 -> Weight Fuel (body fixed)/1, Sum/2
  MatrixMultiply/1 -> Sum/1
  Weight_Fuel/1(Weight_Fuel) -> MatrixMultiply1/2
  Weigh_lander/1 -> MatrixMultiply/2
  Sum/1 -> Total Weight/1

== system MAIN_V4/Plant/Forces and Moments/Forces Body Fixed Frame/Fuel Slosh Disturbance (Body Fixed Frame/Forces Slosh ==
  "EA, EAd, EAdd" : Inport
  "EA, EAd, EAdd1" : Inport  Port=2
  Mass Fuel : Inport  Port=3
  Constant : Constant  Value=cmFuel_cmL
  Subsystem1 : Subsystem
  Subsystem2 : Subsystem
  Fx : Outport
  Fy : Outport  Port=2
  wires:
  "EA, EAd, EAdd1"/1 -> Subsystem2/1("EA, EAd, EAdd")  "Pitch"
  Subsystem2/1(Fy) -> Fy/1
  "EA, EAd, EAdd"/1 -> Subsystem1/1("EA, EAd, EAdd")  "Roll"
  Subsystem1/1(Fx) -> Fx/1
  Constant/1 -> Subsystem2/3(Arm Length), Subsystem1/3(Arm Length)
  Mass Fuel/1 -> Subsystem1/2(Mass Fuel), Subsystem2/2(Mass Fuel)

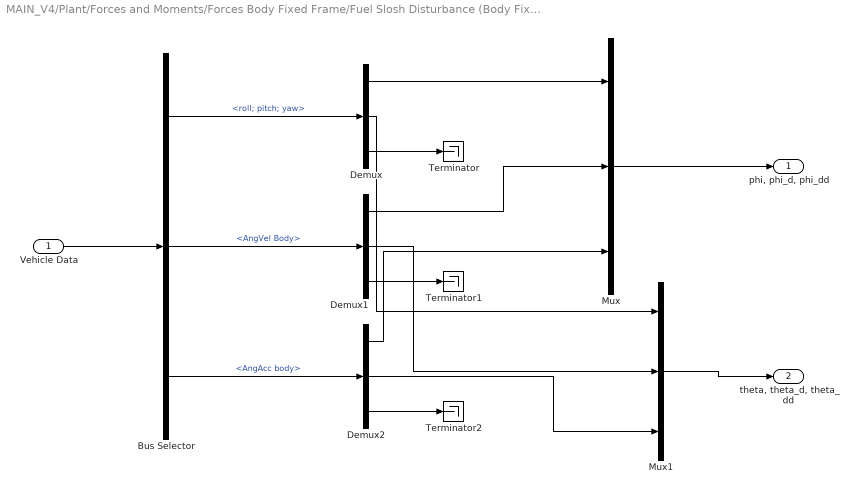
== system MAIN_V4/Plant/Forces and Moments/Forces Body Fixed Frame/Fuel Slosh Disturbance (Body Fixed Frame/Subsystem ==
  Vehicle Data : Inport
  Bus Selector : BusSelector  OutputSignals=roll; pitch; yaw,AngVel Body,AngAcc body
  Demux : Demux  Outputs=3
  Demux1 : Demux  Outputs=3
  Demux2 : Demux  Outputs=3
  Mux : Mux  Inputs=3
  Mux1 : Mux  Inputs=3
  Terminator : Terminator
  Terminator1 : Terminator
  Terminator2 : Terminator
  "phi, phi_d, phi_dd" : Outport
  "theta, theta_d, theta_dd" : Outport  Port=2
  wires:
  Bus Selector/1 -> Demux/1  "<roll; pitch; yaw>"
  Bus Selector/2 -> Demux1/1  "<AngVel Body>"
  Bus Selector/3 -> Demux2/1  "<AngAcc body>"
  Demux/1 -> Mux/1
  Demux1/1 -> Mux/2
  Demux2/1 -> Mux/3
  Mux/1 -> "phi, phi_d, phi_dd"/1
  Demux/2 -> Mux1/1
  Demux1/2 -> Mux1/2
  Demux2/2 -> Mux1/3
  Demux/3 -> Terminator/1
  Demux1/3 -> Terminator1/1
  Demux2/3 -> Terminator2/1
  Mux1/1 -> "theta, theta_d, theta_dd"/1
  Vehicle Data/1 -> Bus Selector/1

== system MAIN_V4/Plant/Forces and Moments/Forces Body Fixed Frame/Weight (Body Fixed Frame)/Weight_Fuel ==
  mass_Fuel : Inport
  Constant : Constant  Value=0
  Gain : Gain  Gain=g
  Mux : Mux  Inputs=3
  Weight_Fuel : Outport
  wires:
  Constant/1 -> Mux/2, Mux/1
  mass_Fuel/1 -> Gain/1
  Mux/1 -> Weight_Fuel/1
  Gain/1 -> Mux/3

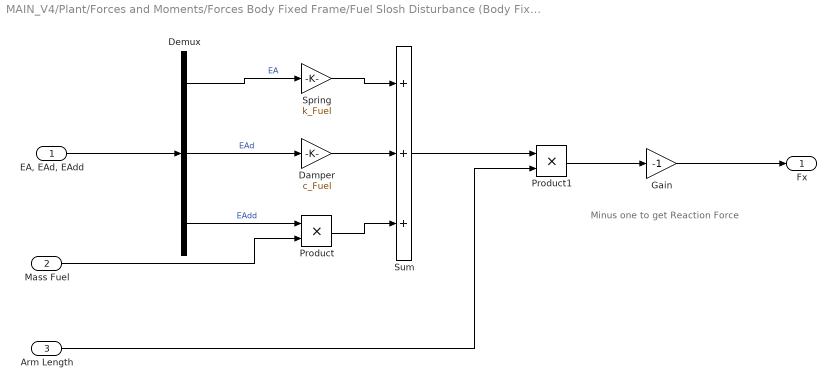
== system MAIN_V4/Plant/Forces and Moments/Forces Body Fixed Frame/Fuel Slosh Disturbance (Body Fixed Frame/Forces Slosh/Subsystem1 ==
  note: Minus one to get Reaction Force
  "EA, EAd, EAdd" : Inport
  Mass Fuel : Inport  Port=2
  Arm Length : Inport  Port=3
  Damper : Gain  Gain=c_Fuel
  Demux : Demux  Outputs=3
  Gain : Gain  Gain=-1
  Product : Product
  Product1 : Product
  Spring : Gain  Gain=k_Fuel
  Sum : Sum  Inputs=+++
  Fx : Outport
  wires:
  Demux/1 -> Spring/1  "EA"
  Demux/2 -> Damper/1  "EAd"
  Demux/3 -> Product/1  "EAdd"
  Mass Fuel/1 -> Product/2
  Product/1 -> Sum/3
  Damper/1 -> Sum/2
  Spring/1 -> Sum/1
  "EA, EAd, EAdd"/1 -> Demux/1
  Sum/1 -> Product1/1
  Arm Length/1 -> Product1/2
  Product1/1 -> Gain/1
  Gain/1 -> Fx/1

== system MAIN_V4/Plant/Forces and Moments/Forces Body Fixed Frame/Fuel Slosh Disturbance (Body Fixed Frame/Forces Slosh/Subsystem2 ==
  note: Minus one to get Reaction Force
  "EA, EAd, EAdd" : Inport
  Mass Fuel : Inport  Port=2
  Arm Length : Inport  Port=3
  Damper : Gain  Gain=c_Fuel
  Demux : Demux  Outputs=3
  Gain : Gain  Gain=-1
  Product : Product
  Product1 : Product
  Spring : Gain  Gain=k_Fuel
  Sum : Sum  Inputs=+++
  Fy : Outport
  wires:
  Demux/1 -> Spring/1  "EA"
  Demux/2 -> Damper/1  "EAd"
  Demux/3 -> Product/1  "EAdd"
  Mass Fuel/1 -> Product/2
  Product/1 -> Sum/3
  Damper/1 -> Sum/2
  Spring/1 -> Sum/1
  "EA, EAd, EAdd"/1 -> Demux/1
  Sum/1 -> Product1/1
  Arm Length/1 -> Product1/2
  Product1/1 -> Gain/1
  Gain/1 -> Fy/1

== matlab function MAIN_V4/Visuals/Coordinate Transforms1/Generalized Principle Axis and Angle of Rotation ==
  data: VRVec output; RotMat input
function VRVec  = fcn(RotMat)
% Rotation algorithms obtained form "Spacecraft Dynamics & Control (ARO
% 4090 text) pg 21 
phi = acos((trace(RotMat) -  1)/2); % eq 1.27
A = 1/(sin(phi)) * [RotMat(2,3) - RotMat(3,2)
                    RotMat(3,1) - RotMat(1,3)
                    RotMat(1,2) - RotMat(2,1)]; % eq 1.28
VRVec = [A;phi];

== matlab function MAIN_V4/Visuals/Coordinate Transforms/Generalized Principle Axis and Angle of Rotation ==
  data: VRVec output; RotMat input
function VRVec  = fcn(RotMat)
% Rotation algorithms obtained form "Spacecraft Dynamics & Control (ARO
% 4090 text) pg 21 
phi = acos((trace(RotMat) -  1)/2); % eq 1.27
A = 1/(sin(phi)) * [RotMat(2,3) - RotMat(3,2)
                    RotMat(3,1) - RotMat(1,3)
                    RotMat(1,2) - RotMat(2,1)]; % eq 1.28
VRVec = [A;phi];

== matlab function MAIN_V4/Visuals/Coordinate Transforms/NED Euler to VR Euler ==
  data: eu input; C output
function C = fcn(eu)
psi = eu(1); % FIrst rotation about NEDbody Fixed x
theta = eu(2); % Second rot about NEd Body fixed y
phi = eu(3); % Second rotation about NedBody Fixed Z

alpha =  -psi; % First rot about VR Body Fixed
beta = theta; % Second rotation about VR Body Fixed
gamm = -phi; % Thirst rot about VR Body fixed
 
Cz = [cos(alpha)  sin(alpha) 0
      -sin(alpha) cos(alpha) 0
      0           0          1];
Cx = [1 0         0
      0 cos(beta)  sin(beta)
      0 -sin(beta) cos(beta)];
Cy = [cos(gamm) 0 -sin(gamm)
      0         1 0
      sin(gamm) 0 cos(gamm)];
C = Cy * Cx * Cz;

== matlab function MAIN_V4/Visuals/Coordinate Transforms1/NED Euler to VR Euler ==
  data: eu input; C output
function C = fcn(eu)
psi = eu(1); % FIrst rotation about NEDbody Fixed x
theta = eu(2); % Second rot about NEd Body fixed y
phi = eu(3); % Second rotation about NedBody Fixed Z

alpha =  -psi; % First rot about VR Body Fixed
beta = theta; % Second rotation about VR Body Fixed
gamm = -phi; % Thirst rot about VR Body fixed
 
Cz = [cos(alpha)  sin(alpha) 0
      -sin(alpha) cos(alpha) 0
      0           0          1];
Cx = [1 0         0
      0 cos(beta)  sin(beta)
      0 -sin(beta) cos(beta)];
Cy = [cos(gamm) 0 -sin(gamm)
      0         1 0
      sin(gamm) 0 cos(gamm)];
C = Cy * Cx * Cz;
